simulink model "irep_force_central"  (Simulink 7.5)
settings: Solver=ode3  StartTime=0.0  StopTime=inf  FixedStep=dt  RelTol=1e-3
InitFcn:
  | IREPOLD_DEPENDENCY
  | init_omni
  | init_filters
  | init_telemanipulation
  | init_parker_xyz
  | init_magnetic_tracker
  | init_loadcell
  | init_scopes
  | init_homing
  | init_force_control
  | init_force_sensing
  | ATI_Init_gamma
undefined symbols (not defined in the file): A, ATI_torque_convert_to_Nmm, dt, dt_trakstar, filter_coeffs_ATI, filter_coeffs_ATI_bias, inv_T, irep_parameters_right, N_ATI, N_ATI_bias, N_trakstar, r, statics_param, trakstar_filter_coeffs
libraries: xpclib x30, simulink x2, dspswit3 x2, xpcmeasurementcomputinglib x1, dspsigops x1
settings Model: Creator=Andrea  LastModifiedBy=Long  BufferReuse=off
settings OptimizationCC: BlockReduction=off  OptimizeBlockIOStorage=off  BufferReuse=off  ExpressionFolding=off  LocalBlockOutputs=off  OptimizeModelRefInitCode=on
settings DebuggingCC: MultiTaskCondExecSysMsg=warning  MultiTaskRateTransMsg=warning  StrictBusMsg=Warning
settings HardwareCC: ProdIntDivRoundTo=Zero  ProdEndianess=LittleEndian  ProdHWDeviceType=Generic->32-bit x86 compatible
settings RTWCC: SystemTargetFile=xpctargetert.tlc  TemplateMakefile=xpc_ert_tmf  Description=xPC Target (ERT)  ProcessScript=xpctargetert_make_rtw_hook  RTWCompilerOptimization=On
settings xpcTargetERTCC: TargetFcnLib=ansi_tfl_table_tmw.mat  TargetFunctionLibrary=ANSI_C  UtilityFuncGeneration=Auto  ERTMultiwordTypeDef=System defined  ERTCodeCoverageTool=None  ERTMultiwordLength=256  MultiwordLength=2048  GenerateFullHeader=on  GenerateSampleERTMain=off  GenerateTestInterfaces=off  IsPILTarget=off  ModelReferenceCompliant=on  ParMdlRefBuildCompliant=off  CompOptLevelCompliant=on  IncludeMdlTerminateFcn=on  GeneratePreprocessorConditionals=Disable all  CombineOutputUpdateFcns=off  SuppressErrorStatus=off  ERTFirstTimeCompliant=off  IncludeFileDelimiter=Auto  ERTCustomFileBanners=off  SupportAbsoluteTime=on  LogVarNameModifier=rt_  MatFileLogging=on  MultiInstanceERTCode=off  SupportNonFinite=on  SupportComplex=on  PurelyIntegerCode=off  SupportContinuousTime=on  SupportNonInlinedSFcns=on  SupportVariableSizeSignals=off  EnableShiftOperators=on  ParenthesesLevel=Nominal  PortableWordSizes=off  ModelStepFunctionPrototypeControlCompliant=off  CPPClassGenCompliant=off  AutosarCompliant=off  GenerateASAP2=off  ExtModeTransport=0  ExtModeStaticAlloc=off  ExtModeStaticAllocSize=1000000  ExtModeTesting=off  InlinedParameterPlacement=NonHierarchical  TargetOS=BareBoardExample  MultiInstanceErrorCode=Error  RateGroupingCode=on  RootIOFormat=Individual arguments  CoverageDialogOpen=off  ERTFilePackagingFormat=Modular  PreserveExpressionOrder=off  PreserveIfCondition=off  ConvertIfToSwitch=off  PreserveExternInFcnDecls=on  EnableUserReplacementTypes=off  MemSecPackage=--- None ---  MemSecDataConstants=Default  MemSecDataIO=Default  MemSecDataInternal=Default  MemSecDataParameters=Default  MemSecFuncInitTerm=Default  MemSecFuncExecute=Default  GRTInterface=on  GlobalDataDefinition=Auto  GlobalDataReference=Auto  ModuleNamingRule=Unspecified  ERTSrcFileBannerTemplate=ert_code_template.cgt  ERTHdrFileBannerTemplate=ert_code_template.cgt  ERTDataSrcFileTemplate=ert_code_template.cgt  ERTDataHdrFileTemplate=ert_code_template.cgt  ERTCustomFileTemplate=example_file_process.tlc  SignalDisplayLevel=10  ParamTuneLevel=10  InitialValueSource=Model  RTWCAPISignals=off  RTWCAPIParams=off  RTWCAPIStates=off  GenerateErtSFunction=off  RL32ModeModifier=Real-Time  ExtMode=on  ExtModeMexFile=ext_xpc  ExtModeIntrfLevel=Level2 - Open  ExtModeArmWhenConnect=off  RL32LogTETModifier=on  RL32LogBufSizeModifier=100000  RL32IRQSourceModifier=Timer  xPCIRQSourceBoard=None/Other  xPCIOIRQSlot=-1  xpcObjCom=off  xPCGenerateASAP2=off  xPCGenerateXML=off  RL32ObjectName=tg  xPCisDownloadable=off  xPCisDefaultEnv=on  xPCisModelTimeout=on  xPCModelTimeoutSecs=5  xpcDblBuff=off  xPCLoadParamSetFile=off

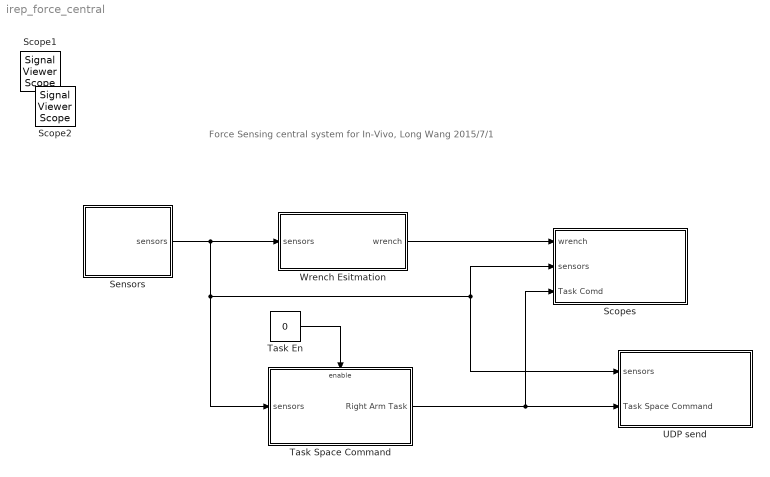
== system irep_force_central ==
  note: Force Sensing central system for In-Vivo, Long Wang 2015/7/1
  Scopes : Subsystem
  Sensors : Subsystem
  Task En : Constant  Value=0  OutDataType=fixdt(1, 16)  OutScaling=2^0
  Task Space Command : Subsystem  TreatAsAtomicUnit=on
  UDP send : Subsystem
  Wrench Esitmation : Subsystem
  Scope1 : SignalViewerScope  IOType=viewer  RefreshTime=0.035000
  Scope2 : SignalViewerScope  IOType=viewer  RefreshTime=0.035000
  wires:
  Sensors/1(sensors) -> Wrench Esitmation/1(sensors), Scopes/2(sensors), UDP send/1(sensors), Task Space Command/1(sensors)
  Wrench Esitmation/1(wrench) -> Scopes/1(wrench)
  Task En/1 -> Task Space Command/Enable
  Task Space Command/1(Right Arm Task) -> UDP send/2(Task Space Command), Scopes/3(Task Comd)

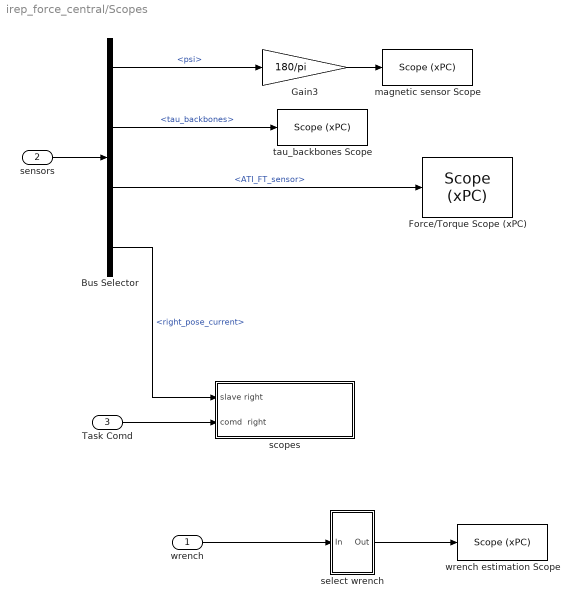
== system irep_force_central/Scopes ==
  wrench : Inport  OutDataType=fixdt(1, 16)  OutScaling=2^0
  sensors : Inport  Port=2  OutDataType=fixdt(1, 16)  OutScaling=2^0
  Task Comd : Inport  Port=3  OutDataType=fixdt(1, 16)  OutScaling=2^0
  Bus Selector : BusSelector  OutputSignals=magnetic_tracker.psi,tau_backbones,ATI_FT_sensor,right_pose_current
  "Force/Torque Scope (xPC) " : xpclib/Misc./Scope (xPC)   SystemSampleTime=-1  scopeno=7  scopetype=Target  autostart=on  viewmode=Numerical  formatstr=scope_format_ATI_wrench  grid=on  ylimits=[0,0]  nosamples=Scope_Samples  noprepostsamples=0  interleave=1  triggermode=FreeRun  triggersignal=1  triggerlevel=0.0  triggerslope=Either  triggerscope=1  triggersample=0  filename=data.dat  mode=Lazy  writesize=512  autorestart=off  dynamicfilemode=off  maxwritefilesize=512*1024^2
  Gain3 : Gain  Gain=180/pi  ParameterDataType=fixdt(1, 16)  ParameterScaling=2^0  OutDataType=fixdt(1, 16)  OutScaling=2^0
  magnetic sensor Scope : xpclib/Misc./Scope (xPC)   SystemSampleTime=-1  scopeno=6  scopetype=Host  autostart=on  viewmode=Numerical  formatstr=scope_format_megnetic_psi  grid=on  ylimits=[0,0]  nosamples=25  noprepostsamples=0  interleave=1  triggermode=FreeRun  triggersignal=1  triggerlevel=0.0  triggerslope=Either  triggerscope=1  triggersample=0  filename=data.dat  mode=Lazy  writesize=512  autorestart=off  dynamicfilemode=off  maxwritefilesize=512*1024^2
  scopes : Subsystem
  select wrench : Subsystem
  tau_backbones Scope : xpclib/Misc./Scope (xPC)   SystemSampleTime=-1  scopeno=4  scopetype=Host  autostart=on  viewmode=Numerical  formatstr=scope_format_tau_backbones  grid=on  ylimits=[0,0]  nosamples=25  noprepostsamples=0  interleave=1  triggermode=FreeRun  triggersignal=1  triggerlevel=0.0  triggerslope=Either  triggerscope=1  triggersample=0  filename=data.dat  mode=Lazy  writesize=512  autorestart=off  dynamicfilemode=off  maxwritefilesize=512*1024^2
  wrench estimation Scope : xpclib/Misc./Scope (xPC)   SystemSampleTime=-1  scopeno=1  scopetype=Host  autostart=on  viewmode=Numerical  formatstr=scope_format_wrench_est_right_arm  grid=on  ylimits=[0,0]  nosamples=25  noprepostsamples=0  interleave=1  triggermode=FreeRun  triggersignal=1  triggerlevel=0.0  triggerslope=Either  triggerscope=1  triggersample=0  filename=data.dat  mode=Lazy  writesize=512  autorestart=off  dynamicfilemode=off  maxwritefilesize=512*1024^2
  wires:
  sensors/1 -> Bus Selector/1
  Gain3/1 -> magnetic sensor Scope/1
  Bus Selector/1 -> Gain3/1  "<psi>"
  Bus Selector/2 -> tau_backbones Scope/1  "<tau_backbones>"
  Bus Selector/3 -> "Force/Torque Scope (xPC) "/1  "<ATI_FT_sensor>"
  wrench/1 -> select wrench/1(In)
  select wrench/1(Out) -> wrench estimation Scope/1
  Bus Selector/4 -> scopes/1(slave right)  "<right_pose_current>"
  Task Comd/1 -> scopes/2(comd  right)

== system irep_force_central/Sensors ==
  ATI Force Torque Sensor : Subsystem
  Bus Creator : BusCreator
  IREP current Pose : Subsystem
  Magnetic Tracker 125 Hz : Subsystem  TreatAsAtomicUnit=on
      mask Display: %image(imread('trakSTAR.jpg'));
  Receive tau_backbones : Subsystem
  sensors : Outport
  wires:
  Receive tau_backbones/1(tau_backbones) -> Bus Creator/2  "tau_backbones"
  ATI Force Torque Sensor/1(Out1) -> Bus Creator/3  "ATI_FT_sensor"
  Magnetic Tracker 125 Hz/1(TrakStar) -> Bus Creator/1  "magnetic_tracker"
  Bus Creator/1 -> sensors/1
  IREP current Pose/1(Right) -> Bus Creator/4  "right_pose_current"

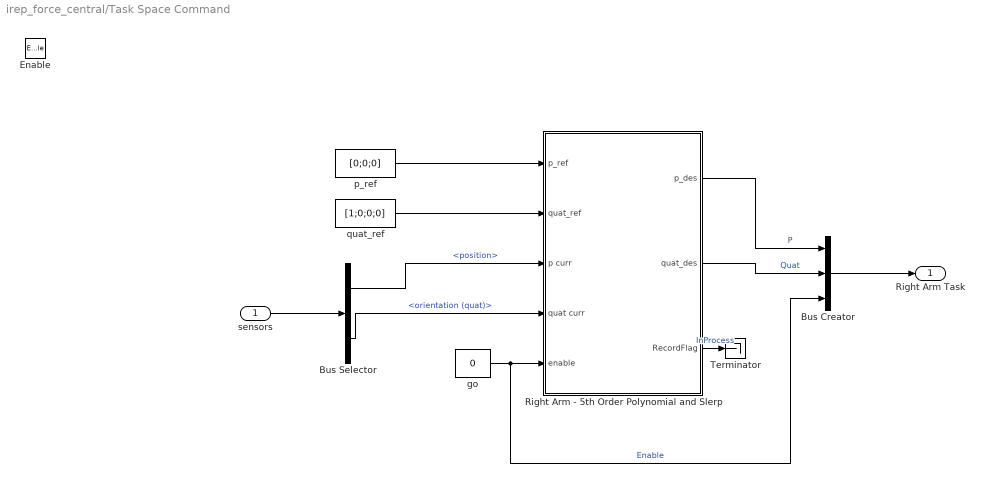
== system irep_force_central/Task Space Command ==
  sensors : Inport
  Enable : EnablePort  StatesWhenEnabling=reset
  Bus Creator : BusCreator  Inputs=3
  Bus Selector : BusSelector  OutputSignals=right_pose_current.position,right_pose_current.orientation (quat)
  Right Arm - 5th Order Polynomial and Slerp : Subsystem
  Terminator : Terminator
  go : Constant  Value=0
  p_ref : Constant  Value=[0;0;0]
  quat_ref : Constant  Value=[1;0;0;0]
  Right Arm Task : Outport  InitialOutput=zeros(9,1)
  wires:
  sensors/1 -> Bus Selector/1
  p_ref/1 -> Right Arm - 5th Order Polynomial and Slerp/1(p_ref)
  Bus Selector/1 -> Right Arm - 5th Order Polynomial and Slerp/3(p curr)  "<position>"
  Bus Selector/2 -> Right Arm - 5th Order Polynomial and Slerp/4(quat curr)  "<orientation (quat)>"
  Right Arm - 5th Order Polynomial and Slerp/1(p_des) -> Bus Creator/1  "P"
  Right Arm - 5th Order Polynomial and Slerp/2(quat_des) -> Bus Creator/2  "Quat"
  Bus Creator/1 -> Right Arm Task/1
  quat_ref/1 -> Right Arm - 5th Order Polynomial and Slerp/2(quat_ref)
  go/1 -> Right Arm - 5th Order Polynomial and Slerp/5(enable), Bus Creator/3  "Enable"
  Right Arm - 5th Order Polynomial and Slerp/3(RecordFlag) -> Terminator/1  "InProcess"

== system irep_force_central/UDP send ==
  sensors : Inport  OutDataType=fixdt(1, 16)  OutScaling=2^0
  Task Space Command : Inport  Port=2  OutDataType=fixdt(1, 16)  OutScaling=2^0
  Bus Selector : BusSelector  OutputSignals=ATI_FT_sensor
  Force UDP Send : Subsystem
  Rate Transition : RateTransition  OutPortSampleTime=dt_UDP_send
  Task Space UDP Send : Subsystem
  wires:
  sensors/1 -> Bus Selector/1
  Bus Selector/1 -> Rate Transition/1  "<ATI_FT_sensor>"
  Rate Transition/1 -> Force UDP Send/1(In1)
  Task Space Command/1 -> Task Space UDP Send/1(In1)

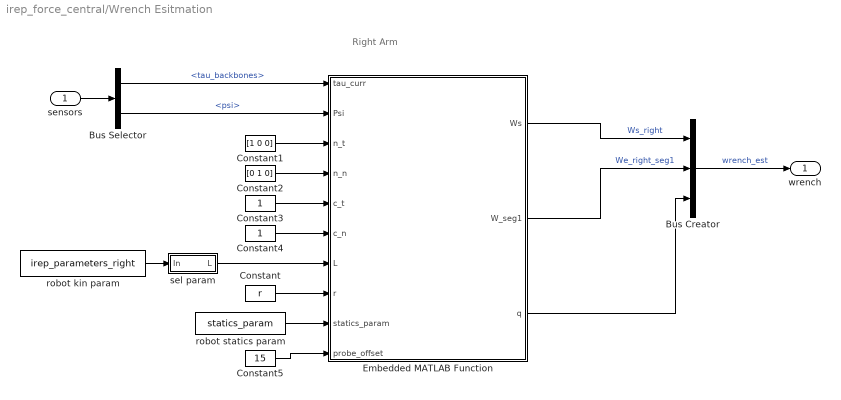
== system irep_force_central/Wrench Esitmation ==
  note: Right Arm
  sensors : Inport
  Bus Creator : BusCreator  Inputs=3
  Bus Selector : BusSelector  OutputSignals=tau_backbones,magnetic_tracker.psi
  Constant : Constant  Value=r  OutDataType=fixdt(1, 16)  OutScaling=2^0
  Constant1 : Constant  Value=[1 0 0]  OutDataType=fixdt(1, 16)  OutScaling=2^0
  Constant2 : Constant  Value=[0 1 0]  OutDataType=fixdt(1, 16)  OutScaling=2^0
  Constant3 : Constant  OutDataType=fixdt(1, 16)  OutScaling=2^0
  Constant4 : Constant  OutDataType=fixdt(1, 16)  OutScaling=2^0
  Constant5 : Constant  Value=15  OutDataType=fixdt(1, 16)  OutScaling=2^0
  Embedded MATLAB Function : Stateflow chart  TreatAsAtomicUnit=on
  robot kin param : Constant  Value=irep_parameters_right  OutDataType=fixdt(1, 16)  OutScaling=2^0
  robot statics param : Constant  Value=statics_param  OutDataType=fixdt(1, 16)  OutScaling=2^0
  sel param : Subsystem
  wrench : Outport
  wires:
  Constant/1 -> Embedded MATLAB Function/8(r)
  Constant1/1 -> Embedded MATLAB Function/3(n_t)
  Constant2/1 -> Embedded MATLAB Function/4(n_n)
  Constant3/1 -> Embedded MATLAB Function/5(c_t)
  Constant4/1 -> Embedded MATLAB Function/6(c_n)
  robot kin param/1 -> sel param/1(In)
  sel param/1(L) -> Embedded MATLAB Function/7(L)
  robot statics param/1 -> Embedded MATLAB Function/9(statics_param)
  Constant5/1 -> Embedded MATLAB Function/10(probe_offset)
  sensors/1 -> Bus Selector/1
  Bus Selector/1 -> Embedded MATLAB Function/1(tau_curr)  "<tau_backbones>"
  Bus Selector/2 -> Embedded MATLAB Function/2(Psi)  "<psi>"
  Embedded MATLAB Function/1(Ws) -> Bus Creator/1  "Ws_right"
  Embedded MATLAB Function/2(W_seg1) -> Bus Creator/2  "We_right_seg1"
  Bus Creator/1 -> wrench/1  "wrench_est"
  Embedded MATLAB Function/3(q) -> Bus Creator/3

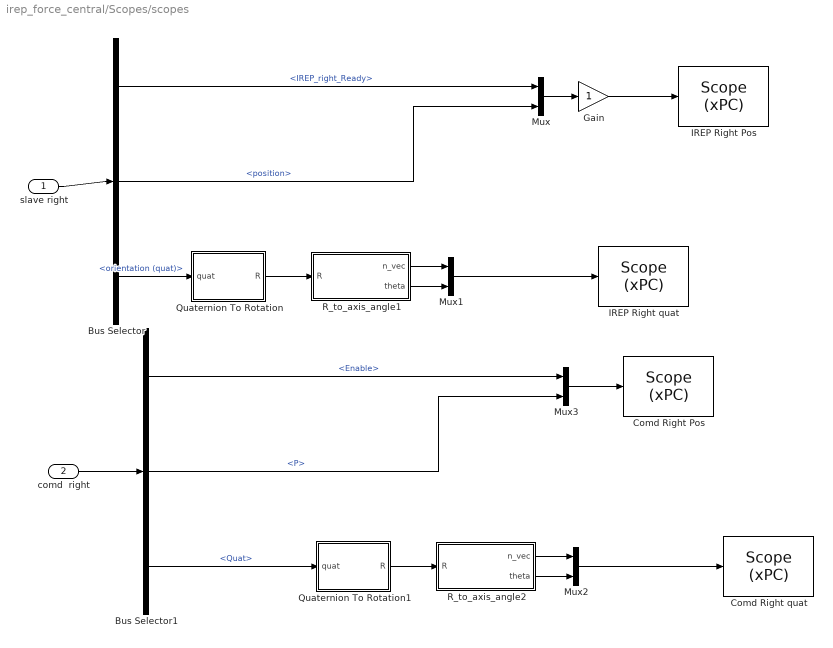
== system irep_force_central/Scopes/scopes ==
  slave right : Inport
  comd  right : Inport  Port=2
  Bus Selector : BusSelector  OutputSignals=IREP_right_Ready,position,orientation (quat)
  Bus Selector1 : BusSelector  OutputSignals=Enable,P,Quat
  Comd Right Pos : xpclib/Misc./Scope (xPC)   SystemSampleTime=-1  scopeno=10  scopetype=Target  autostart=on  viewmode=Numerical  formatstr=scope_format_Comd_R_pos  grid=on  ylimits=[0,0]  nosamples=25  noprepostsamples=0  interleave=1  triggermode=FreeRun  triggersignal=1  triggerlevel=0.0  triggerslope=Either  triggerscope=1  triggersample=0  filename=data.dat  mode=Lazy  writesize=512  autorestart=off  dynamicfilemode=off  maxwritefilesize=512*1024^2
  Comd Right quat : xpclib/Misc./Scope (xPC)   SystemSampleTime=-1  scopeno=8  scopetype=Target  autostart=on  viewmode=Numerical  formatstr=scope_format_Comd_R_quat  grid=on  ylimits=[0,0]  nosamples=25  noprepostsamples=0  interleave=1  triggermode=FreeRun  triggersignal=1  triggerlevel=0.0  triggerslope=Either  triggerscope=1  triggersample=0  filename=data.dat  mode=Lazy  writesize=512  autorestart=off  dynamicfilemode=off  maxwritefilesize=512*1024^2
  Gain : Gain  ParameterDataType=fixdt(1, 16)  ParameterScaling=2^0  OutDataType=fixdt(1, 16)  OutScaling=2^0
  IREP Right Pos : xpclib/Misc./Scope (xPC)   SystemSampleTime=-1  scopeno=2  scopetype=Target  autostart=on  viewmode=Numerical  formatstr=scope_format_IREP_R_pos  grid=on  ylimits=[0,0]  nosamples=25  noprepostsamples=0  interleave=1  triggermode=FreeRun  triggersignal=1  triggerlevel=0.0  triggerslope=Either  triggerscope=1  triggersample=0  filename=data.dat  mode=Lazy  writesize=512  autorestart=off  dynamicfilemode=off  maxwritefilesize=512*1024^2
  IREP Right quat : xpclib/Misc./Scope (xPC)   SystemSampleTime=-1  scopeno=3  scopetype=Target  autostart=on  viewmode=Numerical  formatstr=scope_format_IREP_R_quat  grid=on  ylimits=[0,0]  nosamples=25  noprepostsamples=0  interleave=1  triggermode=FreeRun  triggersignal=1  triggerlevel=0.0  triggerslope=Either  triggerscope=1  triggersample=0  filename=data.dat  mode=Lazy  writesize=512  autorestart=off  dynamicfilemode=off  maxwritefilesize=512*1024^2
  Mux{,1..3} (4 alike) : Mux  Inputs=2
  Quaternion To Rotation : Stateflow chart  TreatAsAtomicUnit=on
  Quaternion To Rotation1 : Stateflow chart  TreatAsAtomicUnit=on
  R_to_axis_angle1 : Stateflow chart  TreatAsAtomicUnit=on
  R_to_axis_angle2 : Stateflow chart  TreatAsAtomicUnit=on
  wires:
  slave right/1 -> Bus Selector/1
  Quaternion To Rotation/1(R) -> R_to_axis_angle1/1(R)
  R_to_axis_angle1/1(n_vec) -> Mux1/1
  R_to_axis_angle1/2(theta) -> Mux1/2
  Bus Selector/1 -> Mux/1  "<IREP_right_Ready>"
  Bus Selector/3 -> Quaternion To Rotation/1(quat)  "<orientation (quat)>"
  Bus Selector/2 -> Mux/2  "<position>"
  Mux/1 -> Gain/1
  Mux1/1 -> IREP Right quat/1
  comd  right/1 -> Bus Selector1/1
  Quaternion To Rotation1/1(R) -> R_to_axis_angle2/1(R)
  R_to_axis_angle2/1(n_vec) -> Mux2/1
  R_to_axis_angle2/2(theta) -> Mux2/2
  Mux2/1 -> Comd Right quat/1
  Bus Selector1/3 -> Quaternion To Rotation1/1(quat)  "<Quat>"
  Bus Selector1/1 -> Mux3/1  "<Enable>"
  Bus Selector1/2 -> Mux3/2  "<P>"
  Mux3/1 -> Comd Right Pos/1
  Gain/1 -> IREP Right Pos/1

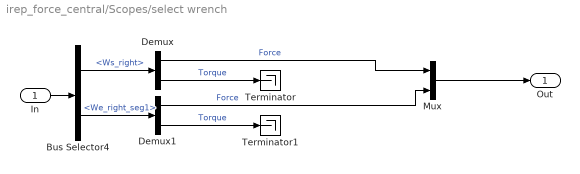
== system irep_force_central/Scopes/select wrench ==
  In : Inport
  Bus Selector4 : BusSelector  OutputSignals=Ws_right,We_right_seg1
  Demux : Demux  Outputs=[3,3]
  Demux1 : Demux  Outputs=[3,3]
  Mux : Mux  Inputs=2
  Terminator : Terminator
  Terminator1 : Terminator
  Out : Outport
  wires:
  Bus Selector4/1 -> Demux/1  "<Ws_right>"
  Bus Selector4/2 -> Demux1/1  "<We_right_seg1>"
  Demux/2 -> Terminator/1  "Torque"
  Demux1/2 -> Terminator1/1  "Torque"
  Demux/1 -> Mux/1  "Force"
  Demux1/1 -> Mux/2  "Force"
  Mux/1 -> Out/1
  In/1 -> Bus Selector4/1

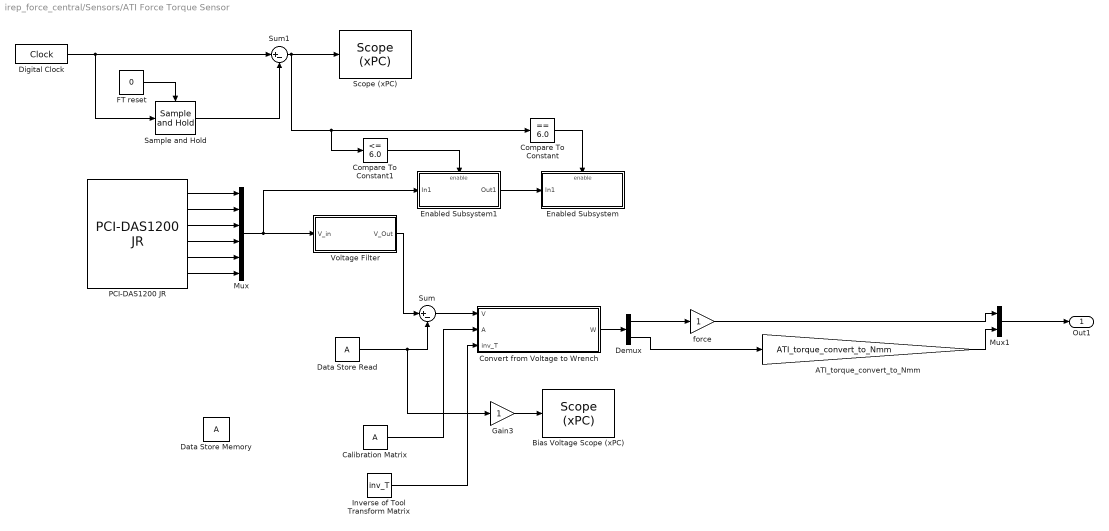
== system irep_force_central/Sensors/ATI Force Torque Sensor ==
  ATI_torque_convert_to_Nmm : Gain  Gain=ATI_torque_convert_to_Nmm
  Bias Voltage Scope (xPC) : xpclib/Misc./Scope (xPC)   SystemSampleTime=-1  scopeno=5  scopetype=Host  autostart=on  viewmode=Numerical  formatstr=Voltage_Vals_format  grid=on  ylimits=[0,0]  nosamples=250  noprepostsamples=0  interleave=1  triggermode=FreeRun  triggersignal=1  triggerlevel=0.0  triggerslope=Either  triggerscope=1  triggersample=0  filename=data.dat  mode=Lazy  writesize=512  autorestart=off  dynamicfilemode=off  maxwritefilesize=512*1024^2
  Calibration Matrix : Constant  Value=A
  Compare To Constant : simulink/Logic and Bit Operations/Compare To Constant  SystemSampleTime=-1  relop===  const=6.0  LogicOutDataTypeMode=uint8  ZeroCross=off
  Compare To Constant1 : simulink/Logic and Bit Operations/Compare To Constant  SystemSampleTime=-1  relop=<=  const=6.0  LogicOutDataTypeMode=uint8  ZeroCross=off
  "Convert from Voltage to Wrench " : Stateflow chart  TreatAsAtomicUnit=on
  Data Store Memory : DataStoreMemory  DataStoreName=A  ReadBeforeWriteMsg=warning  WriteAfterWriteMsg=warning  WriteAfterReadMsg=warning  InitialValue=[0;0;0;0;0;0]
  Data Store Read : DataStoreRead  DataStoreName=A  SampleTime=0
  Demux : Demux  Outputs=2
  Digital Clock : DigitalClock  SampleTime=dt
  Enabled Subsystem : Subsystem  TreatAsAtomicUnit=on
  Enabled Subsystem1 : Subsystem  TreatAsAtomicUnit=on
  FT reset : Constant  Value=0  OutDataType=fixdt(1, 16)  OutScaling=2^0
  Gain3 : Gain
  Inverse of Tool Transform Matrix : Constant  Value=inv_T  VectorParams1D=off
  Mux : Mux  Inputs=6
  Mux1 : Mux  Inputs=2
  "PCI-DAS1200 JR " : xpcmeasurementcomputinglib/A//D/PCI-DAS1200 JR   channel=6  range=+-10V  mux=Single-ended (16 channels)  sampletime=dt  slot=[2 12]
  Sample and Hold : dspsigops/Sample and Hold  SystemSampleTime=-1  trig=Rising edge  initCond=0  latchinput=off
  "Scope (xPC) " : xpclib/Misc./Scope (xPC)   SystemSampleTime=-1  scopeno=9  scopetype=Host  autostart=on  viewmode=Numerical  formatstr='%15.6f'  grid=on  ylimits=[0,0]  nosamples=25  noprepostsamples=0  interleave=1  triggermode=FreeRun  triggersignal=1  triggerlevel=0.0  triggerslope=Either  triggerscope=1  triggersample=0  filename=data.dat  mode=Lazy  writesize=512  autorestart=off  dynamicfilemode=off  maxwritefilesize=512*1024^2
  Sum : Sum  Inputs=|+-
  Sum1 : Sum  Inputs=|+-  OutDataType=fixdt(1, 16)  OutScaling=2^0
  Voltage Filter : Subsystem
  force : Gain
  Out1 : Outport  OutDataType=fixdt(1, 16)  OutScaling=2^0
  wires:
  Mux/1 -> Voltage Filter/1(V_in), Enabled Subsystem1/1(In1)
  Calibration Matrix/1 -> "Convert from Voltage to Wrench "/2(A)
  Inverse of Tool Transform Matrix/1 -> "Convert from Voltage to Wrench "/3(inv_T)
  Sum/1 -> "Convert from Voltage to Wrench "/1(V)
  Voltage Filter/1(V_Out) -> Sum/1
  Data Store Read/1 -> Sum/2, Gain3/1
  Enabled Subsystem1/1(Out1) -> Enabled Subsystem/1(In1)
  Compare To Constant/1 -> Enabled Subsystem/Enable
  Gain3/1 -> Bias Voltage Scope (xPC)/1
  Compare To Constant1/1 -> Enabled Subsystem1/Enable
  "PCI-DAS1200 JR "/1 -> Mux/1
  "PCI-DAS1200 JR "/2 -> Mux/2
  "PCI-DAS1200 JR "/3 -> Mux/3
  "PCI-DAS1200 JR "/4 -> Mux/4
  "PCI-DAS1200 JR "/5 -> Mux/5
  "PCI-DAS1200 JR "/6 -> Mux/6
  Digital Clock/1 -> Sum1/1, Sample and Hold/1
  Sum1/1 -> Compare To Constant/1, Compare To Constant1/1, "Scope (xPC) "/1
  Sample and Hold/1 -> Sum1/2
  FT reset/1 -> Sample and Hold/Trigger
  Demux/1 -> force/1
  Demux/2 -> ATI_torque_convert_to_Nmm/1
  ATI_torque_convert_to_Nmm/1 -> Mux1/2
  force/1 -> Mux1/1
  Mux1/1 -> Out1/1
  "Convert from Voltage to Wrench "/1(W) -> Demux/1

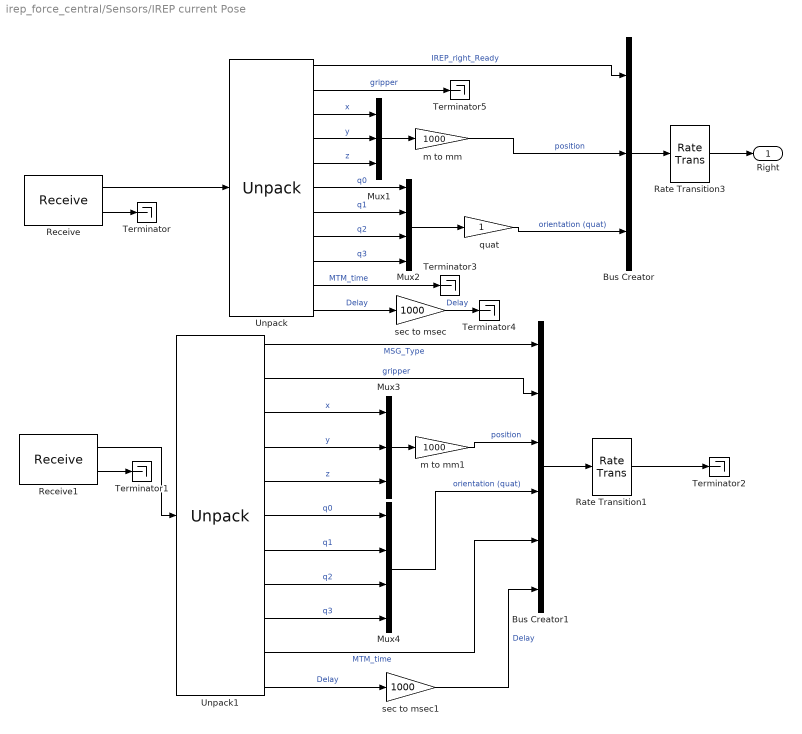
== system irep_force_central/Sensors/IREP current Pose ==
  Bus Creator : BusCreator  Inputs=3
  Bus Creator1 : BusCreator  Inputs=6
  Mux1 : Mux  Inputs=3
  Mux2 : Mux
  Mux3 : Mux  Inputs=3
  Mux4 : Mux
  Rate Transition1 : RateTransition  OutPortSampleTime=dt
  Rate Transition3 : RateTransition  OutPortSampleTime=dt
  Receive : xpclib/UDP/Receive  ipAddress=0.0.0.0  ipPort=10005  width=8*11  vblLen=on  sampletime=dt_omni
  Receive1 : xpclib/UDP/Receive  ipAddress=0.0.0.0  ipPort=10004  width=8*11  vblLen=on  sampletime=dt_omni
  Terminator{,1..5} (6 alike) : Terminator
  Unpack : xpclib/UDP/Unpack  dimensions={1,1,1,1,1,1,1,1,1,1,1}  datatypes={'double' 'double' 'double' 'double' 'double' 'double' 'double' 'double' 'double' 'double' 'double'}  byteAlign=1
  Unpack1 : xpclib/UDP/Unpack  dimensions={1,1,1,1,1,1,1,1,1,1,1}  datatypes={'double' 'double' 'double' 'double' 'double' 'double' 'double' 'double' 'double' 'double' 'double'}  byteAlign=1
  m to mm : Gain  Gain=1000  ParameterDataType=fixdt(1, 16)  ParameterScaling=2^0  OutDataType=fixdt(1, 16)  OutScaling=2^0
  m to mm1 : Gain  Gain=1000  ParameterDataType=fixdt(1, 16)  ParameterScaling=2^0  OutDataType=fixdt(1, 16)  OutScaling=2^0
  quat : Gain  ParameterDataType=fixdt(1, 16)  ParameterScaling=2^0  OutDataType=fixdt(1, 16)  OutScaling=2^0
  sec to msec : Gain  Gain=1000  ParameterDataType=fixdt(1, 16)  ParameterScaling=2^0  OutDataType=fixdt(1, 16)  OutScaling=2^0
  sec to msec1 : Gain  Gain=1000  ParameterDataType=fixdt(1, 16)  ParameterScaling=2^0  OutDataType=fixdt(1, 16)  OutScaling=2^0
  Right : Outport
  wires:
  Bus Creator/1 -> Rate Transition3/1
  Receive/2 -> Terminator/1
  Receive/1 -> Unpack/1
  Bus Creator1/1 -> Rate Transition1/1
  Rate Transition1/1 -> Terminator2/1
  Receive1/2 -> Terminator1/1
  Receive1/1 -> Unpack1/1
  Unpack/9 -> Mux2/4  "q3"
  Unpack/8 -> Mux2/3  "q2"
  Unpack/7 -> Mux2/2  "q1"
  Unpack/6 -> Mux2/1  "q0"
  Unpack/5 -> Mux1/3  "z"
  Unpack/4 -> Mux1/2  "y"
  Unpack/3 -> Mux1/1  "x"
  Unpack1/6 -> Mux4/1  "q0"
  Unpack1/7 -> Mux4/2  "q1"
  Unpack1/8 -> Mux4/3  "q2"
  Unpack1/9 -> Mux4/4  "q3"
  Unpack1/3 -> Mux3/1  "x"
  Unpack1/4 -> Mux3/2  "y"
  Unpack1/5 -> Mux3/3  "z"
  Mux1/1 -> m to mm/1
  Unpack/1 -> Bus Creator/1  "IREP_right_Ready"
  Mux4/1 -> Bus Creator1/4  "orientation (quat)"
  Mux3/1 -> m to mm1/1
  Unpack1/2 -> Bus Creator1/2  "gripper"
  Unpack1/1 -> Bus Creator1/1  "MSG_Type"
  m to mm1/1 -> Bus Creator1/3  "position"
  Unpack/11 -> sec to msec/1  "Delay"
  Unpack1/10 -> Bus Creator1/5  "MTM_time"
  Unpack1/11 -> sec to msec1/1  "Delay"
  sec to msec1/1 -> Bus Creator1/6  "Delay"
  Unpack/10 -> Terminator3/1  "MTM_time"
  sec to msec/1 -> Terminator4/1  "Delay"
  Unpack/2 -> Terminator5/1  "gripper"
  m to mm/1 -> Bus Creator/2  "position"
  Mux2/1 -> quat/1
  Rate Transition3/1 -> Right/1
  quat/1 -> Bus Creator/3  "orientation (quat)"

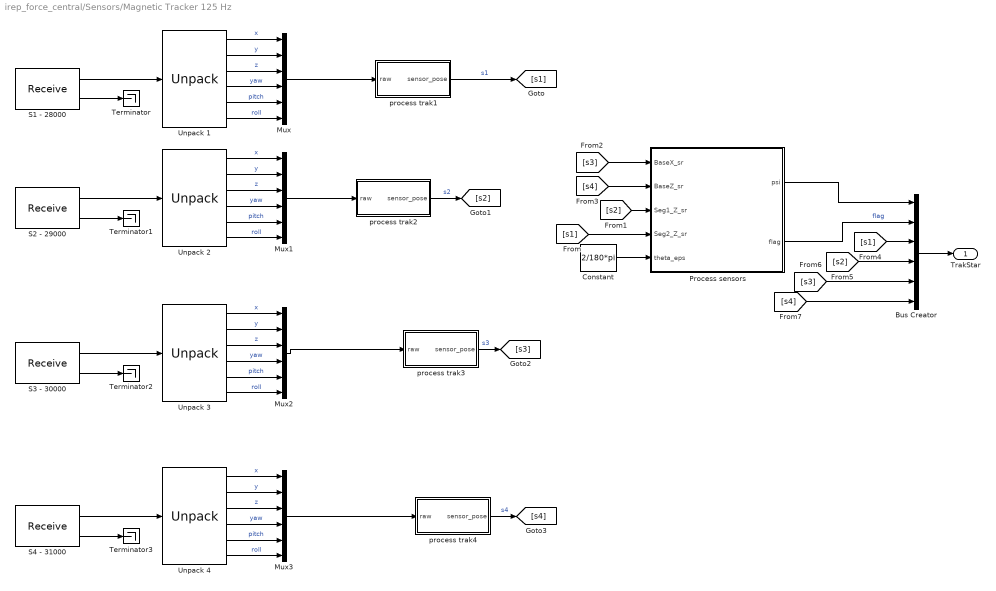
== system irep_force_central/Sensors/Magnetic Tracker 125 Hz ==
  Bus Creator : BusCreator  Inputs=6
  Constant : Constant  Value=2/180*pi  OutDataType=fixdt(1, 16)  OutScaling=2^0
  Mux{,1..3} (4 alike) : Mux  Inputs=6
  Process sensors : Stateflow chart  TreatAsAtomicUnit=on
  S1 - 28000 : xpclib/UDP/Receive  ipAddress=0.0.0.0  ipPort=28000  width=48  vblLen=on  sampletime=dt_trakstar
  S2 - 29000 : xpclib/UDP/Receive  ipAddress=0.0.0.0  ipPort=29000  width=48  vblLen=on  sampletime=dt_trakstar
  S3 - 30000 : xpclib/UDP/Receive  ipAddress=0.0.0.0  ipPort=30000  width=48  vblLen=on  sampletime=dt_trakstar
  S4 - 31000 : xpclib/UDP/Receive  ipAddress=0.0.0.0  ipPort=31000  width=48  vblLen=on  sampletime=dt_trakstar
  Terminator{,1..3} (4 alike) : Terminator
  Unpack {1..4} (4 alike) : xpclib/UDP/Unpack  dimensions={1,1,1,1,1,1}  datatypes={'double' 'double' 'double' 'double' 'double' 'double'}  byteAlign=1
  process trak1 : Subsystem
  process trak2 : Subsystem
  process trak3 : Subsystem
  process trak4 : Subsystem
  TrakStar : Outport  OutDataType=fixdt(1, 16)  OutScaling=2^0
  wires:
  S1 - 28000/1 -> Unpack 1/1
  S1 - 28000/2 -> Terminator/1
  Unpack 1/1 -> Mux/1  "x"
  Unpack 1/2 -> Mux/2  "y"
  Unpack 1/3 -> Mux/3  "z"
  Unpack 1/4 -> Mux/4  "yaw"
  Unpack 1/5 -> Mux/5  "pitch"
  Unpack 1/6 -> Mux/6  "roll"
  Mux/1 -> process trak1/1(raw)
  S2 - 29000/1 -> Unpack 2/1
  S2 - 29000/2 -> Terminator1/1
  Unpack 2/1 -> Mux1/1  "x"
  Unpack 2/2 -> Mux1/2  "y"
  Unpack 2/3 -> Mux1/3  "z"
  Unpack 2/4 -> Mux1/4  "yaw"
  Unpack 2/5 -> Mux1/5  "pitch"
  Unpack 2/6 -> Mux1/6  "roll"
  Mux1/1 -> process trak2/1(raw)
  Bus Creator/1 -> TrakStar/1
  S3 - 30000/1 -> Unpack 3/1
  S3 - 30000/2 -> Terminator2/1
  Unpack 3/1 -> Mux2/1  "x"
  Unpack 3/2 -> Mux2/2  "y"
  Unpack 3/3 -> Mux2/3  "z"
  Unpack 3/4 -> Mux2/4  "yaw"
  Unpack 3/5 -> Mux2/5  "pitch"
  Unpack 3/6 -> Mux2/6  "roll"
  Mux2/1 -> process trak3/1(raw)
  S4 - 31000/1 -> Unpack 4/1
  S4 - 31000/2 -> Terminator3/1
  Unpack 4/1 -> Mux3/1  "x"
  Unpack 4/2 -> Mux3/2  "y"
  Unpack 4/3 -> Mux3/3  "z"
  Unpack 4/4 -> Mux3/4  "yaw"
  Unpack 4/5 -> Mux3/5  "pitch"
  Unpack 4/6 -> Mux3/6  "roll"
  Mux3/1 -> process trak4/1(raw)
  Constant/1 -> Process sensors/5(theta_eps)
  Process sensors/1(psi) -> Bus Creator/1
  process trak1/1(sensor_pose) -> [s1]  "s1"
  [s1] -> Process sensors/4(Seg2_Z_sr)
  process trak2/1(sensor_pose) -> [s2]  "s2"
  [s2] -> Process sensors/3(Seg1_Z_sr)
  process trak3/1(sensor_pose) -> [s3]  "s3"
  [s3] -> Process sensors/1(BaseX_sr)
  process trak4/1(sensor_pose) -> [s4]  "s4"
  [s4] -> Process sensors/2(BaseZ_sr)
  [s1] -> Bus Creator/3
  [s2] -> Bus Creator/4
  [s3] -> Bus Creator/5
  [s4] -> Bus Creator/6
  Process sensors/2(flag) -> Bus Creator/2  "flag"

== system irep_force_central/Sensors/Receive tau_backbones ==
  Mux : Mux  Inputs=8
  Receive : xpclib/UDP/Receive  ipAddress=0.0.0.0  ipPort=25000  width=64  vblLen=off  sampletime=dt
  Terminator : Terminator
  Unpack : xpclib/UDP/Unpack  dimensions={1,1,1,1,1,1,1,1}  datatypes={'double' 'double' 'double' 'double' 'double' 'double' 'double' 'double'}  byteAlign=1
  tau_backbones : Outport
  wires:
  Receive/2 -> Terminator/1
  Receive/1 -> Unpack/1
  Unpack/1 -> Mux/1  "seg1.bb1"
  Unpack/2 -> Mux/2  "seg1.bb2"
  Unpack/3 -> Mux/3  "seg1.bb3"
  Unpack/4 -> Mux/4  "seg1.bb4"
  Unpack/5 -> Mux/5  "seg2.bb1"
  Unpack/6 -> Mux/6  "seg2.bb2"
  Unpack/7 -> Mux/7  "seg2.bb3"
  Unpack/8 -> Mux/8  "seg2.bb4"
  Mux/1 -> tau_backbones/1

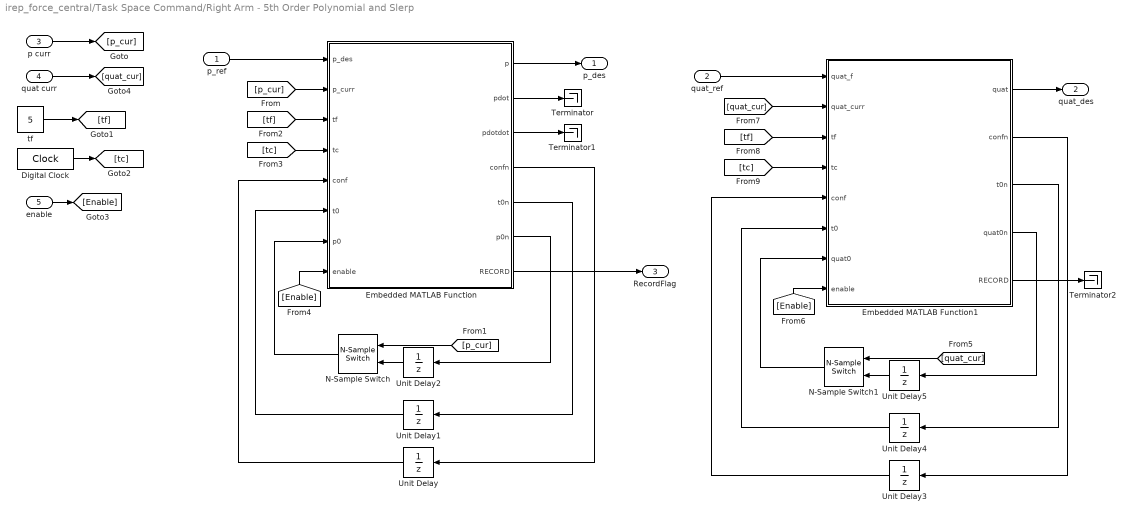
== system irep_force_central/Task Space Command/Right Arm - 5th Order Polynomial and Slerp ==
  p_ref : Inport
  quat_ref : Inport  Port=2
  p curr : Inport  Port=3
  quat curr : Inport  Port=4
  enable : Inport  Port=5
  Digital Clock : DigitalClock  SampleTime=dt
  Embedded MATLAB Function : Stateflow chart  TreatAsAtomicUnit=on
  Embedded MATLAB Function1 : Stateflow chart  TreatAsAtomicUnit=on
  N-Sample Switch : dspswit3/N-Sample Switch  SystemSampleTime=-1  N=1  reset=off  TriggerType=Rising edge  Ts=dt
  N-Sample Switch1 : dspswit3/N-Sample Switch  SystemSampleTime=-1  N=1  reset=off  TriggerType=Rising edge  Ts=dt
  Terminator : Terminator
  Terminator1 : Terminator
  Terminator2 : Terminator
  Unit Delay{,1..4} (5 alike) : UnitDelay  SampleTime=dt
  Unit Delay5 : UnitDelay  X0=[1;0;0;0]  SampleTime=dt
  tf : Constant  Value=5  SampleTime=dt
  p_des : Outport
  quat_des : Outport  Port=2
  RecordFlag : Outport  Port=3
  wires:
  Embedded MATLAB Function/4(confn) -> Unit Delay/1
  Unit Delay/1 -> Embedded MATLAB Function/5(conf)
  Embedded MATLAB Function/5(t0n) -> Unit Delay1/1
  Embedded MATLAB Function/6(p0n) -> Unit Delay2/1
  Unit Delay1/1 -> Embedded MATLAB Function/6(t0)
  p_ref/1 -> Embedded MATLAB Function/1(p_des)
  Embedded MATLAB Function/2(pdot) -> Terminator/1
  Embedded MATLAB Function/3(pdotdot) -> Terminator1/1
  N-Sample Switch/1 -> Embedded MATLAB Function/7(p0)
  Unit Delay2/1 -> N-Sample Switch/2
  p curr/1 -> [p_cur]
  [p_cur] -> Embedded MATLAB Function/2(p_curr)
  [p_cur] -> N-Sample Switch/1
  Embedded MATLAB Function/7(RECORD) -> RecordFlag/1
  Embedded MATLAB Function/1(p) -> p_des/1
  tf/1 -> [tf]
  Digital Clock/1 -> [tc]
  [tf] -> Embedded MATLAB Function/3(tf)
  [tc] -> Embedded MATLAB Function/4(tc)
  enable/1 -> [Enable]
  [Enable] -> Embedded MATLAB Function/8(enable)
  quat_ref/1 -> Embedded MATLAB Function1/1(quat_f)
  quat curr/1 -> [quat_cur]
  Embedded MATLAB Function1/3(t0n) -> Unit Delay4/1
  Embedded MATLAB Function1/4(quat0n) -> Unit Delay5/1
  Unit Delay4/1 -> Embedded MATLAB Function1/6(t0)
  N-Sample Switch1/1 -> Embedded MATLAB Function1/7(quat0)
  Unit Delay5/1 -> N-Sample Switch1/2
  [quat_cur] -> N-Sample Switch1/1
  Embedded MATLAB Function1/2(confn) -> Unit Delay3/1
  Unit Delay3/1 -> Embedded MATLAB Function1/5(conf)
  [Enable] -> Embedded MATLAB Function1/8(enable)
  [quat_cur] -> Embedded MATLAB Function1/2(quat_curr)
  [tf] -> Embedded MATLAB Function1/3(tf)
  [tc] -> Embedded MATLAB Function1/4(tc)
  Embedded MATLAB Function1/1(quat) -> quat_des/1
  Embedded MATLAB Function1/5(RECORD) -> Terminator2/1

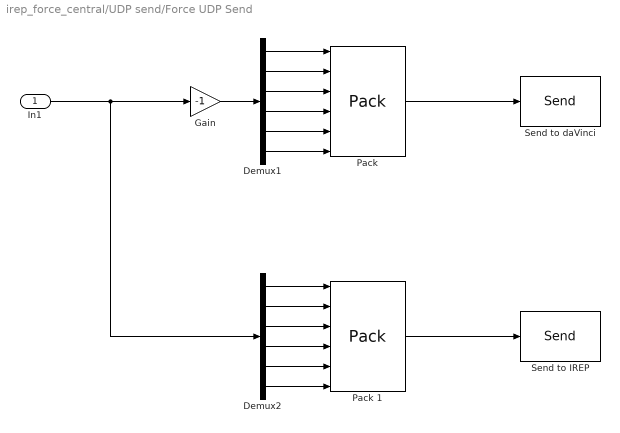
== system irep_force_central/UDP send/Force UDP Send ==
  In1 : Inport
  Demux1 : Demux  Outputs=6
  Demux2 : Demux  Outputs=6
  Gain : Gain  Gain=-1  ParameterDataType=fixdt(1, 16)  ParameterScaling=2^0  OutDataType=fixdt(1, 16)  OutScaling=2^0
  "Pack " : xpclib/UDP/Pack  datatypes={'double' 'double' 'double' 'double' 'double' 'double'}  byteAlign=1
  Pack 1 : xpclib/UDP/Pack  datatypes={'double' 'double' 'double' 'double' 'double' 'double'}  byteAlign=1
  Send to IREP : xpclib/UDP/Send  ipAddress=192.168.1.201  ipPort=20001  localPort=-1  vblLen=off  sampletime=dt_UDP_send
  Send to daVinci : xpclib/UDP/Send  ipAddress=192.168.1.104  ipPort=20001  localPort=-1  vblLen=off  sampletime=dt_UDP_send
  wires:
  In1/1 -> Gain/1, Demux2/1
  Demux1/5 -> "Pack "/5
  Demux1/2 -> "Pack "/2
  Demux1/1 -> "Pack "/1
  Demux1/6 -> "Pack "/6
  Demux1/3 -> "Pack "/3
  Demux1/4 -> "Pack "/4
  "Pack "/1 -> Send to daVinci/1
  Gain/1 -> Demux1/1
  Demux2/5 -> Pack 1/5
  Demux2/2 -> Pack 1/2
  Demux2/1 -> Pack 1/1
  Demux2/3 -> Pack 1/3
  Demux2/4 -> Pack 1/4
  Pack 1/1 -> Send to IREP/1
  Demux2/6 -> Pack 1/6

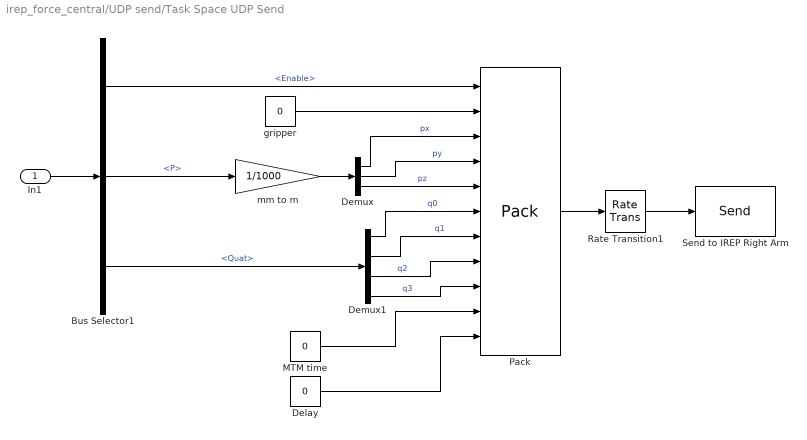
== system irep_force_central/UDP send/Task Space UDP Send ==
  In1 : Inport
  Bus Selector1 : BusSelector  OutputSignals=Enable,P,Quat
  Delay : Constant  Value=0  OutDataType=fixdt(1, 16)  OutScaling=2^0
  Demux : Demux  Outputs=3
  Demux1 : Demux
  MTM time : Constant  Value=0  OutDataType=fixdt(1, 16)  OutScaling=2^0
  "Pack " : xpclib/UDP/Pack  datatypes={'double' 'double' 'double' 'double' 'double' 'double' 'double' 'double' 'double' 'double' 'double'}  byteAlign=1
  Rate Transition1 : RateTransition  OutPortSampleTime=dt_omni
  Send to IREP Right Arm : xpclib/UDP/Send  ipAddress=192.168.1.201  ipPort=10005  localPort=-1  vblLen=off  sampletime=dt_omni
  gripper : Constant  Value=0  OutDataType=fixdt(1, 16)  OutScaling=2^0
  mm to m : Gain  Gain=1/1000  ParameterDataType=fixdt(1, 16)  ParameterScaling=2^0  OutDataType=fixdt(1, 16)  OutScaling=2^0
  wires:
  "Pack "/1 -> Rate Transition1/1
  In1/1 -> Bus Selector1/1
  Bus Selector1/2 -> mm to m/1  "<P>"
  Bus Selector1/1 -> "Pack "/1  "<Enable>"
  gripper/1 -> "Pack "/2
  mm to m/1 -> Demux/1
  Demux/1 -> "Pack "/3  "px"
  Demux/2 -> "Pack "/4  "py"
  Demux/3 -> "Pack "/5  "pz"
  Bus Selector1/3 -> Demux1/1  "<Quat>"
  Demux1/1 -> "Pack "/6  "q0"
  Demux1/2 -> "Pack "/7  "q1"
  Demux1/3 -> "Pack "/8  "q2"
  Demux1/4 -> "Pack "/9  "q3"
  MTM time/1 -> "Pack "/10
  Delay/1 -> "Pack "/11
  Rate Transition1/1 -> Send to IREP Right Arm/1

== system irep_force_central/Wrench Esitmation/sel param ==
  note: irep_parameters_right = [Y_OFFSET;L1r;L2r;p_gripper];
  In : Inport
  Demux : Demux  Outputs=[1,1,1,3]
  Mux1 : Mux  Inputs=2
  Terminator : Terminator
  Terminator1 : Terminator
  L : Outport
  wires:
  In/1 -> Demux/1
  Mux1/1 -> L/1
  Demux/2 -> Mux1/1  "L1"
  Demux/3 -> Mux1/2  "L2"
  Demux/1 -> Terminator/1  "Y_OFFSET"
  Demux/4 -> Terminator1/1  "p_gripper"

== system irep_force_central/Sensors/ATI Force Torque Sensor/Enabled Subsystem ==
  In1 : Inport
  Enable : EnablePort
  Data Store Write : DataStoreWrite  DataStoreName=A  SampleTime=-1
  wires:
  In1/1 -> Data Store Write/1

== system irep_force_central/Sensors/ATI Force Torque Sensor/Enabled Subsystem1 ==
  In1 : Inport
  Enable : EnablePort
  Voltage Filter Bias : Subsystem
  Out1 : Outport
  wires:
  In1/1 -> Voltage Filter Bias/1(V_in)
  Voltage Filter Bias/1(V_Out) -> Out1/1

== system irep_force_central/Sensors/ATI Force Torque Sensor/Voltage Filter ==
  V_in : Inport
  Discrete FIR Filter : DiscreteFir  CoefSource=Input port
  Gain : Gain  Gain=1/N_ATI
  filter_coeffs : Constant  Value=filter_coeffs_ATI
  V_Out : Outport
  wires:
  V_in/1 -> Discrete FIR Filter/1
  Discrete FIR Filter/1 -> Gain/1
  filter_coeffs/1 -> Discrete FIR Filter/2
  Gain/1 -> V_Out/1

== system irep_force_central/Sensors/Magnetic Tracker 125 Hz/process trak1 ==
  raw : Inport
  Filter1 : Subsystem
  Gain : Gain  Gain=[25.4 25.4 25.4 1 1 1]  ParameterDataType=fixdt(1, 16)  ParameterScaling=2^0  OutDataType=fixdt(1, 16)  OutScaling=2^0  SampleTime=dt_trakstar
  trakstar_to_pose : Stateflow chart  TreatAsAtomicUnit=on
  sensor_pose : Outport
  wires:
  Gain/1 -> Filter1/1(in)
  Filter1/1(out) -> trakstar_to_pose/1(u)
  raw/1 -> Gain/1
  trakstar_to_pose/1(sensor) -> sensor_pose/1

== system irep_force_central/Sensors/Magnetic Tracker 125 Hz/process trak2 ==
  raw : Inport
  Filter1 : Subsystem
  Gain : Gain  Gain=[25.4 25.4 25.4 1 1 1]  ParameterDataType=fixdt(1, 16)  ParameterScaling=2^0  OutDataType=fixdt(1, 16)  OutScaling=2^0  SampleTime=dt_trakstar
  trakstar_to_pose : Stateflow chart  TreatAsAtomicUnit=on
  sensor_pose : Outport
  wires:
  trakstar_to_pose/1(sensor) -> sensor_pose/1
  raw/1 -> Gain/1
  Filter1/1(out) -> trakstar_to_pose/1(u)
  Gain/1 -> Filter1/1(in)

== system irep_force_central/Sensors/Magnetic Tracker 125 Hz/process trak3 ==
  raw : Inport
  Filter1 : Subsystem
  Gain : Gain  Gain=[25.4 25.4 25.4 1 1 1]  ParameterDataType=fixdt(1, 16)  ParameterScaling=2^0  OutDataType=fixdt(1, 16)  OutScaling=2^0  SampleTime=dt_trakstar
  trakstar_to_pose : Stateflow chart  TreatAsAtomicUnit=on
  sensor_pose : Outport
  wires:
  Gain/1 -> Filter1/1(in)
  Filter1/1(out) -> trakstar_to_pose/1(u)
  raw/1 -> Gain/1
  trakstar_to_pose/1(sensor) -> sensor_pose/1

== system irep_force_central/Sensors/Magnetic Tracker 125 Hz/process trak4 ==
  raw : Inport
  Filter1 : Subsystem
  Gain : Gain  Gain=[25.4 25.4 25.4 1 1 1]  ParameterDataType=fixdt(1, 16)  ParameterScaling=2^0  OutDataType=fixdt(1, 16)  OutScaling=2^0  SampleTime=dt_trakstar
  trakstar_to_pose : Stateflow chart  TreatAsAtomicUnit=on
  sensor_pose : Outport
  wires:
  trakstar_to_pose/1(sensor) -> sensor_pose/1
  raw/1 -> Gain/1
  Filter1/1(out) -> trakstar_to_pose/1(u)
  Gain/1 -> Filter1/1(in)

== system irep_force_central/Sensors/ATI Force Torque Sensor/Enabled Subsystem1/Voltage Filter Bias ==
  V_in : Inport
  Discrete FIR Filter : DiscreteFir  CoefSource=Input port
  Gain : Gain  Gain=1/N_ATI_bias
  filter_coeffs : Constant  Value=filter_coeffs_ATI_bias
  V_Out : Outport
  wires:
  Gain/1 -> V_Out/1
  filter_coeffs/1 -> Discrete FIR Filter/2
  Discrete FIR Filter/1 -> Gain/1
  V_in/1 -> Discrete FIR Filter/1

== system irep_force_central/Sensors/Magnetic Tracker 125 Hz/process trak1/Filter1 ==
  in : Inport  OutDataType=sfix(16)  OutScaling=2^0
  Discrete FIR Filter : DiscreteFir  CoefSource=Input port  SampleTime=dt_trakstar
  Gain : Gain  Gain=1/N_trakstar  ParameterDataType=sfix(16)  ParameterScaling=2^0  OutDataType=sfix(16)  OutScaling=2^0  SampleTime=dt_trakstar
  trakstar_filter_coeffs : Constant  Value=trakstar_filter_coeffs  OutDataType=sfix(16)  OutScaling=2^0  SampleTime=dt_trakstar
  out : Outport  OutDataType=sfix(16)  OutScaling=2^0
  wires:
  Gain/1 -> out/1
  in/1 -> Discrete FIR Filter/1
  Discrete FIR Filter/1 -> Gain/1
  trakstar_filter_coeffs/1 -> Discrete FIR Filter/2

== system irep_force_central/Sensors/Magnetic Tracker 125 Hz/process trak2/Filter1 ==
  in : Inport  OutDataType=sfix(16)  OutScaling=2^0
  Discrete FIR Filter : DiscreteFir  CoefSource=Input port  SampleTime=dt_trakstar
  Gain : Gain  Gain=1/N_trakstar  ParameterDataType=sfix(16)  ParameterScaling=2^0  OutDataType=sfix(16)  OutScaling=2^0  SampleTime=dt_trakstar
  trakstar_filter_coeffs : Constant  Value=trakstar_filter_coeffs  OutDataType=sfix(16)  OutScaling=2^0  SampleTime=dt_trakstar
  out : Outport  OutDataType=sfix(16)  OutScaling=2^0
  wires:
  trakstar_filter_coeffs/1 -> Discrete FIR Filter/2
  Discrete FIR Filter/1 -> Gain/1
  in/1 -> Discrete FIR Filter/1
  Gain/1 -> out/1

== system irep_force_central/Sensors/Magnetic Tracker 125 Hz/process trak3/Filter1 ==
  in : Inport  OutDataType=sfix(16)  OutScaling=2^0
  Discrete FIR Filter : DiscreteFir  CoefSource=Input port  SampleTime=dt_trakstar
  Gain : Gain  Gain=1/N_trakstar  ParameterDataType=sfix(16)  ParameterScaling=2^0  OutDataType=sfix(16)  OutScaling=2^0  SampleTime=dt_trakstar
  trakstar_filter_coeffs : Constant  Value=trakstar_filter_coeffs  OutDataType=sfix(16)  OutScaling=2^0  SampleTime=dt_trakstar
  out : Outport  OutDataType=sfix(16)  OutScaling=2^0
  wires:
  Gain/1 -> out/1
  in/1 -> Discrete FIR Filter/1
  Discrete FIR Filter/1 -> Gain/1
  trakstar_filter_coeffs/1 -> Discrete FIR Filter/2

== system irep_force_central/Sensors/Magnetic Tracker 125 Hz/process trak4/Filter1 ==
  in : Inport  OutDataType=sfix(16)  OutScaling=2^0
  Discrete FIR Filter : DiscreteFir  CoefSource=Input port  SampleTime=dt_trakstar
  Gain : Gain  Gain=1/N_trakstar  ParameterDataType=sfix(16)  ParameterScaling=2^0  OutDataType=sfix(16)  OutScaling=2^0  SampleTime=dt_trakstar
  trakstar_filter_coeffs : Constant  Value=trakstar_filter_coeffs  OutDataType=sfix(16)  OutScaling=2^0  SampleTime=dt_trakstar
  out : Outport  OutDataType=sfix(16)  OutScaling=2^0
  wires:
  trakstar_filter_coeffs/1 -> Discrete FIR Filter/2
  Discrete FIR Filter/1 -> Gain/1
  in/1 -> Discrete FIR Filter/1
  Gain/1 -> out/1

== matlab function Task Space Command/Right Arm - 5th Order Polynomial and Slerp/Embedded MATLAB Function ==
  data: p output double; p_des input double; p_curr input double; tf input double; tc input double; pdot output double; pdotdot output double; conf input double; confn output double; t0 input double; t0n output double; p0n output double; p0 input double; enable input double; RECORD output double
function [p,pdot,pdotdot,confn,t0n,p0n,RECORD] = fifth_order_p(p_des,p_curr,tf,tc,conf,t0,p0,enable)

n = 3;
RECORD = 0;

if enable == 0                  % Configuration space is not used (pdot = 0). 
    p = p_curr;
    pdotdot = zeros(n,1);
    pdot = zeros(n,1);          % However we do want to record the current 
    confn = 0;                  % position in order to be ready as soon 
    t0n = tc;                   % as the enable becomes 1. 
    p0n = p_curr;
else
    if (p_des-p0)'*(p_des-p0) > 0
        if conf == 0                % conf = 0 means that the 5th order poly 
            p0n = p0;               % is not configured for the desired trajectory.
            t0n = tc;               % Therefore, the block is initialized.
            confn = 1;
            pdot = zeros(n,1);
            p = p0;
            pdotdot = zeros(n,1);
        else
            p0n = p0;
            t0n = t0;
            confn = conf;
            % 5th order polynomial
            a0 = p0;
            a4 = -15*(p_des-p0);
            a3 = -2/3 * a4;
            a5 = -2/5 * a4;
            t = tc-t0;
            tau = t/tf;
            if t < tf
                RECORD = 1;
                p = a0 + a3 * tau^3 + a4 * tau^4 + a5 * tau^5;
                pdot = 3*a3*t^2/tf^3 + 4*a4*t^3/tf^4 + 5*a5*t^4/tf^5;
                pdotdot = 6*a3*t/tf^3 + 12*a4*t^2/tf^4 + 20*a5*t^3/tf^5;
            else
                p = p_des;
                pdot = zeros(n,1);
                pdotdot = zeros(n,1);
                p0n = p_des;
            end
        end
    else
        p = p_des;
        pdot = zeros(n,1);
        pdotdot = zeros(n,1);
        confn = 0;
        p0n = p0;
        t0n = t0;
    end
end
%------------------------------------------------------------------------

== matlab function Sensors/ATI Force Torque Sensor/Convert from Voltage to Wrench  ==
  data: V input double; W output double; A input double; inv_T input double
function W = Convert_Function(V,A,inv_T)%A_vec,p)

W = inv_T*A*V;

== matlab function Task Space Command/Right Arm - 5th Order Polynomial and Slerp/Embedded MATLAB Function1 ==
  data: quat output double; quat_f input double; quat_curr input double; tf input double; tc input double; conf input double; confn output double; t0 input double; t0n output double; quat0n output double; quat0 input double; enable input double; RECORD output double
function [quat,confn,t0n,quat0n,RECORD] = quat_slerp(quat_f,quat_curr,tf,tc,conf,t0,quat0,enable)
%%  modified version of 5th order poly for Slerp
%   
RECORD = 0;
if enable == 0                  % Configuration space is not used (pdot = 0). 
    quat = quat_curr;
    confn = 0;                  % position in order to be ready as soon 
    t0n = tc;                   % as the enable becomes 1. 
    quat0n = quat_curr;
else
    if (quat0'*quat_f)<1
        if conf == 0                % conf = 0 means that the 5th order poly 
            quat0n = quat0;               % is not configured for the desired trajectory.
            t0n = tc;               % Therefore, the block is initialized.
            confn = 1;
            quat = quat0;
        else
            quat0n = quat0;
            t0n = t0;
            confn = conf;
            % Slerp
            t = tc-t0;
            tau = t/tf;
            if t < tf
                RECORD = 1;
                quat = slerp(quat0,quat_f,tau);
            else
                quat = quat_f;
                quat0n = quat_f;
            end
        end
    else
        quat = quat_f;
        confn = 0;
        quat0n = quat0;
        t0n = t0;
    end
end
%------------------------------------------------------------------------

== matlab function Scopes/scopes/Quaternion To Rotation1 ==
  data: quat input double; R output double
function R = fcn(quat)
%#eml
if norm(quat)==0
    quat = [1;0;0;0];
end
R = quat2rot(quat);

== matlab function Scopes/scopes/R_to_axis_angle2 ==
  data: R input double; n_vec output double; theta output double
function [n_vec,theta] = fcn(R)
%#eml
% Axis_angle(R) gives the rotation axis and the rotation angle extracted from rotation matrix R
% Note this function handles singular cases even if theta=0 or theta=180
% degrees, which cause the normal axis equation to become undefined.
% Written by N. Simaan
% Last updated 10/14/2012.

cos_theta=(trace(R)-1)/2;
sin_theta=(1/2)*sqrt((R(3,2)-R(2,3))^2 + (R(1,3)-R(3,1))^2 + (R(2,1)-R(1,2))^2);
theta=atan2(sin_theta,cos_theta);
index=0;
if abs(sin_theta)>1e-6 % before it was 1e-12, Long Wang changed it.
    n_cross=1/(2*sin_theta)*(R-R');
    n_vec=[-n_cross(2,3);n_cross(1,3);-n_cross(1,2)]; %disp('aaa');
    n_vec=n_vec/norm(n_vec);
else
    if cos_theta>0  %this means identity matrix
        n_vec=[0;0;0]; %I choose this arbitrarily to designate the special case for identity matrix
    else  %this is the case where theta is 180 degrees
        nx=sqrt((R(1,1)-cos_theta)/(1-cos_theta));
        ny=sqrt((R(2,2)-cos_theta)/(1-cos_theta));
        nz=sqrt((R(3,3)-cos_theta)/(1-cos_theta));
        
        %%% find the axis that best fits the given rotation matrix
        signs=[[1;1;1],...
               [1;-1;1],...
               [1;-1;-1],...
               [1;1;-1],...
               [-1;1;1],...
               [-1;-1;1],...
               [-1;-1;-1],...
               [-1;1;-1]];
        
        e=zeros(1,8); 
        
        for i=1:1:8
            n_candidate=signs(:,i).*[nx;ny;nz];
            Temp=rotd(n_candidate,theta*180/pi), %rotd takes its input in degrees
            e(1,i)=sum(sum((Temp-R).*(Temp-R)));
        end;    
              e,
        e_min=min(e); %the best fit    
        index=0
        for i=1:1:8  %find the index of the combination that produces the closest rotation
            if e(1,i)==e_min 
                index=i;
                break; 
            end;
        end;
        
        n_vec=signs(:,index).*[nx;ny;nz];
    end
end

== matlab function Scopes/scopes/R_to_axis_angle1 ==
  data: R input double; n_vec output double; theta output double
function [n_vec,theta] = fcn(R)
%#eml
% Axis_angle(R) gives the rotation axis and the rotation angle extracted from rotation matrix R
% Note this function handles singular cases even if theta=0 or theta=180
% degrees, which cause the normal axis equation to become undefined.
% Written by N. Simaan
% Last updated 10/14/2012.

cos_theta=(trace(R)-1)/2;
sin_theta=(1/2)*sqrt((R(3,2)-R(2,3))^2 + (R(1,3)-R(3,1))^2 + (R(2,1)-R(1,2))^2);
theta=atan2(sin_theta,cos_theta);
index=0;
if abs(sin_theta)>1e-6 % before it was 1e-12, Long Wang changed it.
    n_cross=1/(2*sin_theta)*(R-R');
    n_vec=[-n_cross(2,3);n_cross(1,3);-n_cross(1,2)]; %disp('aaa');
    n_vec=n_vec/norm(n_vec);
else
    if cos_theta>0  %this means identity matrix
        n_vec=[0;0;0]; %I choose this arbitrarily to designate the special case for identity matrix
    else  %this is the case where theta is 180 degrees
        nx=sqrt((R(1,1)-cos_theta)/(1-cos_theta));
        ny=sqrt((R(2,2)-cos_theta)/(1-cos_theta));
        nz=sqrt((R(3,3)-cos_theta)/(1-cos_theta));
        
        %%% find the axis that best fits the given rotation matrix
        signs=[[1;1;1],...
               [1;-1;1],...
               [1;-1;-1],...
               [1;1;-1],...
               [-1;1;1],...
               [-1;-1;1],...
               [-1;-1;-1],...
               [-1;1;-1]];
        
        e=zeros(1,8); 
        
        for i=1:1:8
            n_candidate=signs(:,i).*[nx;ny;nz];
            Temp=rotd(n_candidate,theta*180/pi), %rotd takes its input in degrees
            e(1,i)=sum(sum((Temp-R).*(Temp-R)));
        end;    
              e,
        e_min=min(e); %the best fit    
        index=0
        for i=1:1:8  %find the index of the combination that produces the closest rotation
            if e(1,i)==e_min 
                index=i;
                break; 
            end;
        end;
        
        n_vec=signs(:,index).*[nx;ny;nz];
    end
end

== matlab function Scopes/scopes/Quaternion To Rotation ==
  data: quat input double; R output double
function R = fcn(quat)
%#eml
if norm(quat)==0
    quat = [1;0;0;0];
end
R = quat2rot(quat);

== matlab function Sensors/Magnetic Tracker 125 Hz/process trak1/trakstar_to_pose ==
  data: u input double; sensor output double
function sensor= trak2pose(u)
%#eml
%   Frame definitions:
%   tb: the base frame of trakstar
%   n:  the norm (the X axis of trasmitter)
u = round(u*100)/100;
orig_pos = u(1:3);
n_in_tb = RotationMatrix(u(4),[0;0;1])*RotationMatrix(u(5),[0;1;0])*[1;0;0];
sensor = [orig_pos(:);n_in_tb(:)] ;

== matlab function Sensors/Magnetic Tracker 125 Hz/process trak2/trakstar_to_pose ==
  data: u input double; sensor output double
function sensor= trak2pose(u)
%#eml
%   Frame definitions:
%   tb: the base frame of trakstar
%   n:  the norm (the X axis of trasmitter)
u = round(u*100)/100;
orig_pos = u(1:3);
n_in_tb = RotationMatrix(u(4),[0;0;1])*RotationMatrix(u(5),[0;1;0])*[1;0;0];
sensor = [orig_pos(:);n_in_tb(:)] ;

== matlab function Sensors/Magnetic Tracker 125 Hz/process trak3/trakstar_to_pose ==
  data: u input double; sensor output double
function sensor= trak2pose(u)
%#eml
%   Frame definitions:
%   tb: the base frame of trakstar
%   n:  the norm (the X axis of trasmitter)
u = round(u*100)/100;
orig_pos = u(1:3);
n_in_tb = RotationMatrix(u(4),[0;0;1])*RotationMatrix(u(5),[0;1;0])*[1;0;0];
sensor = [orig_pos(:);n_in_tb(:)] ;

== matlab function Sensors/Magnetic Tracker 125 Hz/process trak4/trakstar_to_pose ==
  data: u input double; sensor output double
function sensor= trak2pose(u)
%#eml
%   Frame definitions:
%   tb: the base frame of trakstar
%   n:  the norm (the X axis of trasmitter)
u = round(u*100)/100;
orig_pos = u(1:3);
n_in_tb = RotationMatrix(u(4),[0;0;1])*RotationMatrix(u(5),[0;1;0])*[1;0;0];
sensor = [orig_pos(:);n_in_tb(:)] ;

== matlab function Wrench Esitmation/Embedded MATLAB Function ==
  data: Ws output double; W_seg1 output double; tau_curr input double; Psi input double; n_t input double; n_n input double; c_t input double; c_n input double; L input double; r input double; statics_param input double; probe_offset input double; q output double
function [Ws,W_seg1,q] = fcn(tau_curr,Psi,n_t,n_n,c_t,c_n,L,r,statics_param,probe_offset)
%#eml
q = in_vivo_invkin(Psi,r);
[Ws,W_seg1] = ...
    right_arm_wrench_estimation(tau_curr,...
    q,Psi,...
    n_t,n_n,...
    c_t,c_n,...
    L,r,...
    statics_param,...
    probe_offset);

== matlab function Sensors/Magnetic Tracker 125 Hz/Process sensors ==
  data: BaseX_sr input double; psi output double; BaseZ_sr input double; Seg1_Z_sr input double; Seg2_Z_sr input double; theta_eps input double; flag output double
function [psi,flag] = fcn(BaseX_sr,BaseZ_sr,Seg1_Z_sr,Seg2_Z_sr,theta_eps)
%#eml
[psi_m,flag] = get_psi_measured_2segments(BaseX_sr,BaseZ_sr,Seg1_Z_sr,Seg2_Z_sr,theta_eps);
psi = [pi/3;pi/3;pi/3;pi/3];
